simulink model "DTMF"  (Simulink 7.1)
settings: Solver=VariableStepDiscrete  StartTime=0  StopTime=5  RelTol=1e-3
PreLoadFcn:
  | Framesize=256,Fs=8000
undefined symbols (not defined in the file or in its folder): Fs
libraries: dspddes3 x14, dspobslib x3, dspbuff3 x2, commutil2 x2, dspsigops x1, dsparch3 x1, dspswit3 x1, dspwin32 x1
settings Model: Creator=stuartm  LastModifiedBy=jfaing  ExtModeTrigMode=oneshot  ExtModeArmWhenConnect=off  BufferReuse=off
settings DataIOCC: LimitDataPoints=off  SignalLoggingName=sigsOut
settings OptimizationCC: BlockReduction=off  BooleanDataType=off  OptimizeBlockIOStorage=off  BufferReuse=off  EnforceIntegerDowncast=off  ExpressionFolding=off  FoldNonRolledExpr=off  LocalBlockOutputs=off
settings DebuggingCC: SaveWithParameterizedLinksMsg=none  SignalResolutionControl=TryResolveAllWithWarning  SolverPrmCheckMsg=none  MultiTaskDSMMsg=warning  MultiTaskCondExecSysMsg=none  StrictBusMsg=None
settings HardwareCC: TargetUnknown=on
settings RTWCC: IncludeERTFirstTime=on
settings GRTTargetCC: TargetFcnLib=ansi_tfl_tmw.mat

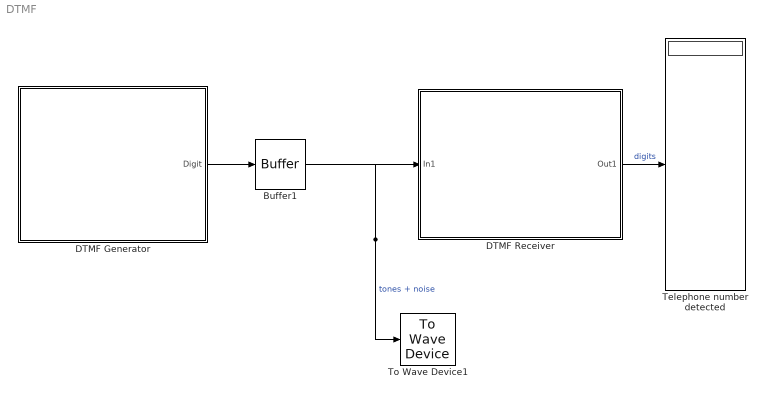
== system DTMF ==
  Buffer1 : dspbuff3/Buffer  N=Framesize  V=0  ic=0
  DTMF Generator : Subsystem
  DTMF Receiver : Subsystem
  Telephone number detected : Display
  To Wave Device1 : dspwin32/To Wave Device  bufDuration=1  determineBufSize=on  userIntBufSize=256  initDelay=0.3  useDefaultDevice=on  userDeviceID=Microsoft RDP Audio Driver  enable24Bit=off
  wires:
  Buffer1/1 -> To Wave Device1/1, DTMF Receiver/1(In1)  "tones + noise"
  DTMF Receiver/1(Out1) -> Telephone number detected/1  "digits"
  DTMF Generator/1(Digit) -> Buffer1/1

== system DTMF/DTMF Generator ==
  Digit to Tone : Subsystem  TreatAsAtomicUnit=on
  Generate telephone number : Subsystem  mask{Number=[1 8 0 0 6 5 3 1 4 1 5], Td=(1/Fs)*256*6}
      mask prompts: Number "Telephone number"; Td "Digit Period (s)"
      mask Display: disp(Number)
  Subtract  1 : Subsystem
  Digit : Outport  OutDataType=sfix(16)  OutScaling=2^0
  wires:
  Generate telephone number/1(Out1) -> Subtract  1/1(In1), Digit to Tone/Enable  "digits"
  Subtract  1/1(Out1) -> Digit to Tone/1(In1)
  Digit to Tone/1(Out1) -> Digit/1

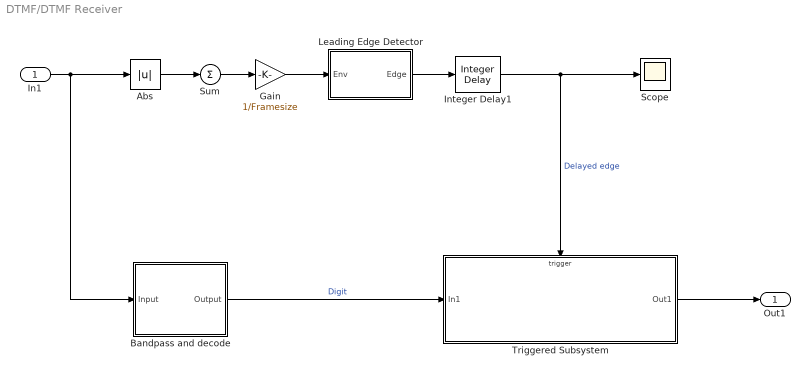
== system DTMF/DTMF Receiver ==
  In1 : Inport  OutDataType=sfix(16)  OutScaling=2^0
  Abs : Abs  SaturateOnIntegerOverflow=on
  Bandpass and decode : Subsystem
  Gain : Gain  Gain=1/Framesize  ParameterDataType=sfix(16)  ParameterScaling=2^0  OutDataType=sfix(16)  OutScaling=2^0  SaturateOnIntegerOverflow=on  OutDataTypeStr=Inherit: Same as input  ParamDataTypeStr=Inherit: Same as input
  Integer Delay1 : dspobslib/Integer Delay  delay=1  ic=0  reset_popup=None
  Leading Edge Detector : Subsystem
  Scope : Scope
  Sum : Sum  Inputs=1  OutDataType=sfix(16)  OutScaling=2^0  SaturateOnIntegerOverflow=on  InputSameDT=on  OutDataTypeStr=Inherit: Same as first input
  Triggered Subsystem : Subsystem  TreatAsAtomicUnit=on
  Out1 : Outport  OutDataType=sfix(16)  OutScaling=2^0
  wires:
  In1/1 -> Abs/1, Bandpass and decode/1(Input)
  Abs/1 -> Sum/1
  Sum/1 -> Gain/1
  Gain/1 -> Leading Edge Detector/1(Env)
  Triggered Subsystem/1(Out1) -> Out1/1
  Integer Delay1/1 -> Scope/1, Triggered Subsystem/Trigger  "Delayed edge"
  Bandpass and decode/1(Output) -> Triggered Subsystem/1(In1)  "Digit"
  Leading Edge Detector/1(Edge) -> Integer Delay1/1

== system DTMF/DTMF Generator/Digit to Tone ==
  In1 : Inport  OutDataType=sfix(16)  OutScaling=2^0
  Enable : EnablePort
  Column Tones 1209Hz 1336Hz 1477Hz : Subsystem
  Column value for digit : Lookup  InputValues=[0 1 2 3 4 5 6 7 8 9 10 11]  Table=[1 0 1 2 0 1 2 0 1 2 0 2]  OutDataType=sfix(16)  OutScaling=2^0  SaturateOnIntegerOverflow=on
  "Row Tones 697Hz 770Hz 852Hz 941Hz " : Subsystem
  Row value for digit : Lookup  InputValues=[0 1 2 3 4 5 6 7 8 9 10 11]  Table=[3 0 0 0 1 1 1 2 2 2 3 3]  OutDataType=sfix(16)  OutScaling=2^0  SaturateOnIntegerOverflow=on
  Sum : Sum  Inputs=|+-  OutDataType=sfix(16)  OutScaling=2^0  SaturateOnIntegerOverflow=on  InputSameDT=on  OutDataTypeStr=Inherit: Same as first input
  Out1 : Outport  OutDataType=sfix(16)  OutScaling=2^0  OutputWhenDisabled=reset  InitialOutput=0
  wires:
  "Row Tones 697Hz 770Hz 852Hz 941Hz "/1(Tone) -> Sum/1
  Column Tones 1209Hz 1336Hz 1477Hz/1(Tone) -> Sum/2
  In1/1 -> Row value for digit/1, Column value for digit/1
  Row value for digit/1 -> "Row Tones 697Hz 770Hz 852Hz 941Hz "/1(Row)
  Column value for digit/1 -> Column Tones 1209Hz 1336Hz 1477Hz/1(Column)
  Sum/1 -> Out1/1

== system DTMF/DTMF Generator/Generate telephone number ==
  Discrete Pulse Generator : DiscretePulseGenerator  SampleTime=Td
  Product : Product  OutDataType=sfix(16)  OutScaling=2^0  SaturateOnIntegerOverflow=on  InputSameDT=on  OutDataTypeStr=Inherit: Same as first input
  Triggered Signal From Workspace1 : dspsigops/Triggered Signal From Workspace  SystemSampleTime=-1  Signal=Number+1  TriggerType=Rising edge  ic=0  SamplesPerFrame=1  OutputAfterFinalValue=Setting to zero
  Out1 : Outport  OutDataType=sfix(16)  OutScaling=2^0
  wires:
  Discrete Pulse Generator/1 -> Product/1, Triggered Signal From Workspace1/Trigger
  Triggered Signal From Workspace1/1 -> Product/2
  Product/1 -> Out1/1

== system DTMF/DTMF Generator/Subtract  1 ==
  In1 : Inport  OutDataType=sfix(16)  OutScaling=2^0
  Constant : Constant  OutDataType=sfix(16)  OutScaling=2^0
  Sum : Sum  Inputs=|+-  OutDataType=sfix(16)  OutScaling=2^0  SaturateOnIntegerOverflow=on  InputSameDT=on  OutDataTypeStr=Inherit: Same as first input
  Out1 : Outport  OutDataType=sfix(16)  OutScaling=2^0
  wires:
  Constant/1 -> Sum/2
  In1/1 -> Sum/1
  Sum/1 -> Out1/1

== system DTMF/DTMF Receiver/Bandpass and decode ==
  Input : Inport  OutDataType=sfix(16)  OutScaling=2^0
  Calculate Digit : Lookup2D  RowIndex=[1:4]  ColumnIndex=[1:3]  Table=[1 2 3;4 5 6;7 8 9;10 0 11]  LookUpMeth=Use Input Nearest  OutDataTypeMode=double  OutDataType=sfix(16)  OutScaling=2^0  OutDataTypeStr=double  SaturateOnIntegerOverflow=on  InputSameDT=on
  Calculate Column : Subsystem
  Calculate Row : Subsystem
  Output : Outport  OutDataType=sfix(16)  OutScaling=2^0
  wires:
  Input/1 -> Calculate Column/1(In1), Calculate Row/1(In1)  "Input Tones"
  Calculate Digit/1 -> Output/1
  Calculate Row/1(Out1) -> Calculate Digit/1
  Calculate Column/1(Out1) -> Calculate Digit/2

== system DTMF/DTMF Receiver/Leading Edge Detector ==
  Env : Inport  OutDataType=sfix(16)  OutScaling=2^0
  Binary To Bipolar : Fcn  Expr=2*u-1
  Constant : Constant  Value=0.5  OutDataType=sfix(16)  OutScaling=2^0
  Direct-Form II Transpose Filter : dsparch3/Direct-Form II Transpose Filter  num=[ones(1,4) -ones(1,4)]  den=1  ic=0
  Edge Detector1 : dspswit3/Edge Detector  SystemSampleTime=-1
  Relational Operator : RelationalOperator  InputSameDT=on
  Rising Edge Start : Fcn  Expr=u>5
  Edge : Outport  OutDataType=sfix(16)  OutScaling=2^0  InitialOutput=0
  wires:
  Edge Detector1/1 -> Edge/1
  Direct-Form II Transpose Filter/1 -> Rising Edge Start/1
  Binary To Bipolar/1 -> Direct-Form II Transpose Filter/1
  Rising Edge Start/1 -> Edge Detector1/1
  Env/1 -> Relational Operator/1
  Constant/1 -> Relational Operator/2
  Relational Operator/1 -> Binary To Bipolar/1

== system DTMF/DTMF Receiver/Triggered Subsystem ==
  In1 : Inport  OutDataType=sfix(16)  OutScaling=2^0
  Trigger : TriggerPort
  Buffer : dspbuff3/Buffer  N=11  V=10  ic=0
  Out1 : Outport  OutDataType=sfix(16)  OutScaling=2^0
  wires:
  In1/1 -> Buffer/1
  Buffer/1 -> Out1/1

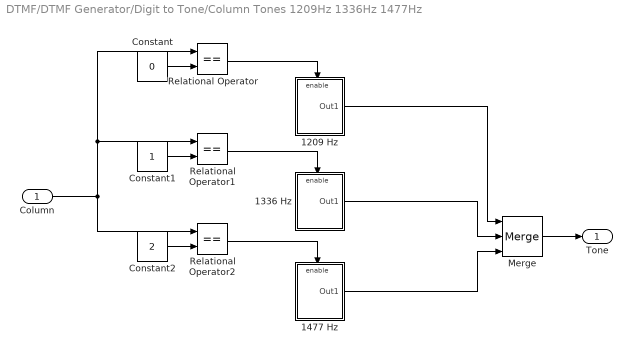
== system DTMF/DTMF Generator/Digit to Tone/Column Tones 1209Hz 1336Hz 1477Hz ==
  Column : Inport  OutDataType=sfix(16)  OutScaling=2^0
  1209 Hz : Subsystem  TreatAsAtomicUnit=on
  1336 Hz : Subsystem  TreatAsAtomicUnit=on
  1477 Hz : Subsystem  TreatAsAtomicUnit=on
  Constant : Constant  Value=0  OutDataType=sfix(16)  OutScaling=2^0
  Constant1 : Constant  OutDataType=sfix(16)  OutScaling=2^0
  Constant2 : Constant  Value=2  OutDataType=sfix(16)  OutScaling=2^0
  Merge : Merge  Inputs=3
  Relational Operator : RelationalOperator  Operator===  InputSameDT=on
  Relational Operator1 : RelationalOperator  Operator===  InputSameDT=on
  Relational Operator2 : RelationalOperator  Operator===  InputSameDT=on
  Tone : Outport  OutDataType=sfix(16)  OutScaling=2^0
  wires:
  Constant2/1 -> Relational Operator2/2
  Constant1/1 -> Relational Operator1/2
  Constant/1 -> Relational Operator/2
  Relational Operator2/1 -> 1477 Hz/Enable
  Relational Operator1/1 -> 1336 Hz/Enable
  Relational Operator/1 -> 1209 Hz/Enable
  Column/1 -> Relational Operator2/1, Relational Operator1/1, Relational Operator/1
  1209 Hz/1(Out1) -> Merge/1
  1336 Hz/1(Out1) -> Merge/2
  1477 Hz/1(Out1) -> Merge/3
  Merge/1 -> Tone/1

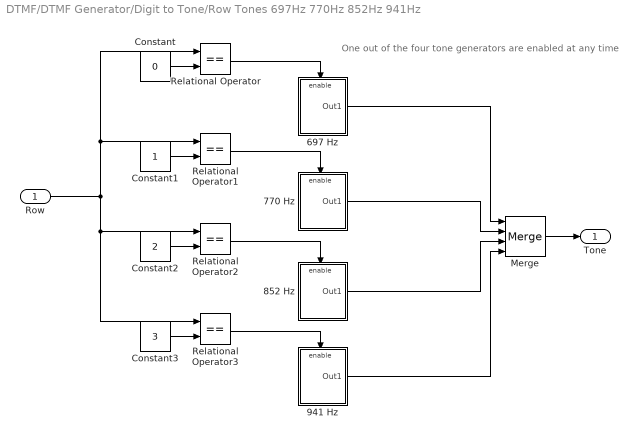
== system DTMF/DTMF Generator/Digit to Tone/Row Tones 697Hz 770Hz 852Hz 941Hz  ==
  note: One out of the four tone generators
      | are enabled at any time
  Row : Inport  OutDataType=sfix(16)  OutScaling=2^0
  697 Hz : Subsystem  TreatAsAtomicUnit=on
  770 Hz : Subsystem  TreatAsAtomicUnit=on
  852 Hz : Subsystem  TreatAsAtomicUnit=on
  941 Hz : Subsystem  TreatAsAtomicUnit=on
  Constant : Constant  Value=0  OutDataType=sfix(16)  OutScaling=2^0
  Constant1 : Constant  OutDataType=sfix(16)  OutScaling=2^0
  Constant2 : Constant  Value=2  OutDataType=sfix(16)  OutScaling=2^0
  Constant3 : Constant  Value=3  OutDataType=sfix(16)  OutScaling=2^0
  Merge : Merge  Inputs=4
  Relational Operator{,1..3} (4 alike) : RelationalOperator  Operator===  InputSameDT=on
  Tone : Outport  OutDataType=sfix(16)  OutScaling=2^0
  wires:
  Constant3/1 -> Relational Operator3/2
  Constant2/1 -> Relational Operator2/2
  Constant1/1 -> Relational Operator1/2
  Constant/1 -> Relational Operator/2
  Relational Operator3/1 -> 941 Hz/Enable
  Relational Operator2/1 -> 852 Hz/Enable
  Relational Operator1/1 -> 770 Hz/Enable
  Relational Operator/1 -> 697 Hz/Enable
  Merge/1 -> Tone/1
  941 Hz/1(Out1) -> Merge/4
  852 Hz/1(Out1) -> Merge/3
  770 Hz/1(Out1) -> Merge/2
  697 Hz/1(Out1) -> Merge/1
  Row/1 -> Relational Operator3/1, Relational Operator2/1, Relational Operator1/1, Relational Operator/1

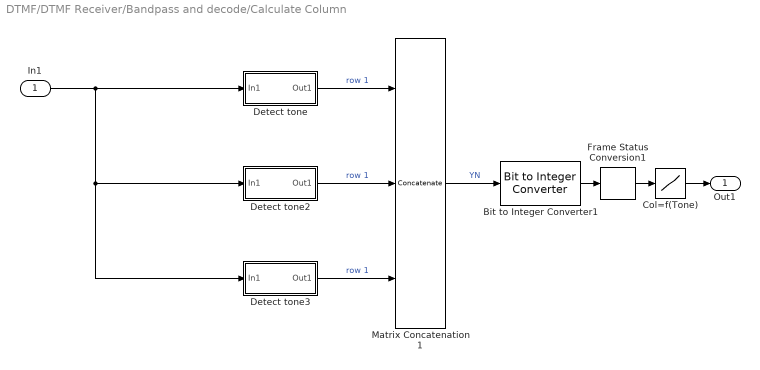
== system DTMF/DTMF Receiver/Bandpass and decode/Calculate Column ==
  In1 : Inport  OutDataType=sfix(16)  OutScaling=2^0
  Bit to Integer Converter1 : commutil2/Bit to Integer Converter  nbits=3  bitOrder=MSB first  signedOutputValues=Unsigned  outDtype=Same as input  outDtypeSigned=Inherit via internal rule
  Col=f(Tone) : Lookup  InputValues=[0:7]  Table=[0 1 2 0 3 0 0 0]  LookUpMeth=Use Input Nearest  OutDataType=sfix(16)  OutScaling=2^0  SaturateOnIntegerOverflow=on
  Detect tone : Subsystem  mask{Fs=Fs, F=1477}
      mask prompts: Fs "Sample Rate (Hz)"; F "Frequency"
      settings: AttributesFormatString=%<F> Hz
  Detect tone2 : Subsystem  mask{Fs=Fs, F=1336}
      mask prompts: Fs "Sample Rate (Hz)"; F "Frequency"
      settings: AttributesFormatString=%<F> Hz
  Detect tone3 : Subsystem  mask{Fs=Fs, F=1209}
      mask prompts: Fs "Sample Rate (Hz)"; F "Frequency"
      settings: AttributesFormatString=%<F> Hz
  Frame Status Conversion1 : dspobslib/Frame Status Conversion  SystemSampleTime=-1  growRefPort=off  outframe=Sample-based
  Matrix Concatenation1 : Concatenate  NumInputs=3  Mode=Multidimensional array
  Out1 : Outport  OutDataType=sfix(16)  OutScaling=2^0
  wires:
  Matrix Concatenation1/1 -> Bit to Integer Converter1/1  "YN"
  Bit to Integer Converter1/1 -> Frame Status Conversion1/1
  Frame Status Conversion1/1 -> Col=f(Tone)/1
  Detect tone/1(Out1) -> Matrix Concatenation1/1  "row 1"
  Detect tone2/1(Out1) -> Matrix Concatenation1/2  "row 1"
  Detect tone3/1(Out1) -> Matrix Concatenation1/3  "row 1"
  In1/1 -> Detect tone2/1(In1), Detect tone3/1(In1), Detect tone/1(In1)
  Col=f(Tone)/1 -> Out1/1

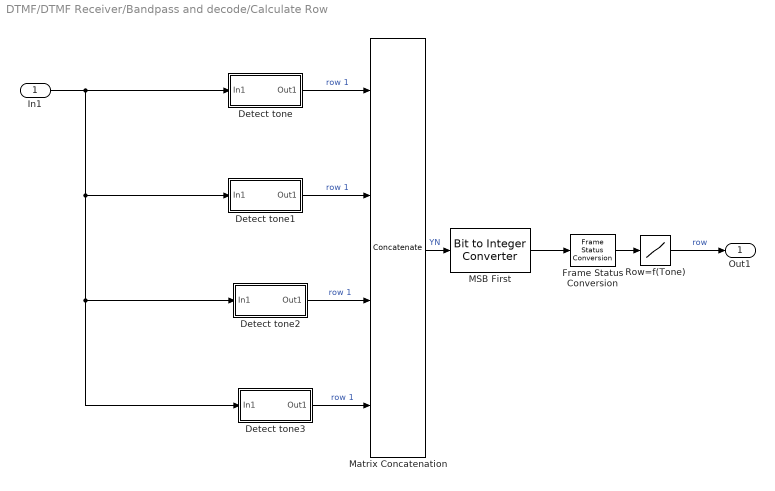
== system DTMF/DTMF Receiver/Bandpass and decode/Calculate Row ==
  In1 : Inport  OutDataType=sfix(16)  OutScaling=2^0
  Detect tone : Subsystem  mask{Fs=Fs, F=941}
      mask prompts: Fs "Sample Rate (Hz)"; F "Frequency"
      settings: AttributesFormatString=%<F> Hz
  Detect tone1 : Subsystem  mask{Fs=Fs, F=852}
      mask prompts: Fs "Sample Rate (Hz)"; F "Frequency"
      settings: AttributesFormatString=%<F> Hz
  Detect tone2 : Subsystem  mask{Fs=Fs, F=770}
      mask prompts: Fs "Sample Rate (Hz)"; F "Frequency"
      settings: AttributesFormatString=%<F> Hz
  Detect tone3 : Subsystem  mask{Fs=Fs, F=697}
      mask prompts: Fs "Sample Rate (Hz)"; F "Frequency"
      settings: AttributesFormatString=%<F> Hz
  Frame Status Conversion : dspobslib/Frame Status Conversion  SystemSampleTime=-1  growRefPort=off  outframe=Sample-based
  MSB First : commutil2/Bit to Integer Converter  nbits=4  bitOrder=MSB first  signedOutputValues=Unsigned  outDtype=Same as input  outDtypeSigned=Inherit via internal rule
  Matrix Concatenation : Concatenate  NumInputs=4  Mode=Multidimensional array
  Row=f(Tone) : Lookup  InputValues=[0:15]  Table=[0 1 2 0 3 0 0 0 4 0 0 0 0 0 0 0]  LookUpMeth=Use Input Nearest  OutDataType=sfix(16)  OutScaling=2^0  SaturateOnIntegerOverflow=on
  Out1 : Outport  OutDataType=sfix(16)  OutScaling=2^0
  wires:
  Detect tone/1(Out1) -> Matrix Concatenation/1  "row 1"
  Matrix Concatenation/1 -> MSB First/1  "YN"
  MSB First/1 -> Frame Status Conversion/1
  Frame Status Conversion/1 -> Row=f(Tone)/1
  Detect tone1/1(Out1) -> Matrix Concatenation/2  "row 1"
  Detect tone2/1(Out1) -> Matrix Concatenation/3  "row 1"
  Detect tone3/1(Out1) -> Matrix Concatenation/4  "row 1"
  In1/1 -> Detect tone/1(In1), Detect tone1/1(In1), Detect tone2/1(In1), Detect tone3/1(In1)
  Row=f(Tone)/1 -> Out1/1  "row"

== system DTMF/DTMF Generator/Digit to Tone/Column Tones 1209Hz 1336Hz 1477Hz/1209 Hz ==
  Enable : EnablePort
  Sine Wave1 : Sin  Frequency=1209*(2*pi)  SampleTime=1/Fs
  Out1 : Outport  OutDataType=sfix(16)  OutScaling=2^0
  wires:
  Sine Wave1/1 -> Out1/1

== system DTMF/DTMF Generator/Digit to Tone/Column Tones 1209Hz 1336Hz 1477Hz/1336 Hz ==
  Enable : EnablePort
  Sine Wave1 : Sin  Frequency=1336*(2*pi)  SampleTime=1/Fs
  Out1 : Outport  OutDataType=sfix(16)  OutScaling=2^0
  wires:
  Sine Wave1/1 -> Out1/1

== system DTMF/DTMF Generator/Digit to Tone/Column Tones 1209Hz 1336Hz 1477Hz/1477 Hz ==
  Enable : EnablePort
  Sine Wave1 : Sin  Frequency=1477*(2*pi)  SampleTime=1/Fs
  Out1 : Outport  OutDataType=sfix(16)  OutScaling=2^0
  wires:
  Sine Wave1/1 -> Out1/1

== system DTMF/DTMF Generator/Digit to Tone/Row Tones 697Hz 770Hz 852Hz 941Hz /697 Hz ==
  Enable : EnablePort
  Sine Wave1 : Sin  Frequency=2*pi*697  SampleTime=1/Fs
  Out1 : Outport  OutDataType=sfix(16)  OutScaling=2^0
  wires:
  Sine Wave1/1 -> Out1/1

== system DTMF/DTMF Generator/Digit to Tone/Row Tones 697Hz 770Hz 852Hz 941Hz /770 Hz ==
  Enable : EnablePort
  Sine Wave1 : Sin  Frequency=2*pi*770  SampleTime=1/Fs
  Out1 : Outport  OutDataType=sfix(16)  OutScaling=2^0
  wires:
  Sine Wave1/1 -> Out1/1

== system DTMF/DTMF Generator/Digit to Tone/Row Tones 697Hz 770Hz 852Hz 941Hz /852 Hz ==
  Enable : EnablePort
  Sine Wave1 : Sin  Frequency=852*(2*pi)  SampleTime=1/Fs
  Out1 : Outport  OutDataType=sfix(16)  OutScaling=2^0
  wires:
  Sine Wave1/1 -> Out1/1

== system DTMF/DTMF Generator/Digit to Tone/Row Tones 697Hz 770Hz 852Hz 941Hz /941 Hz ==
  Enable : EnablePort
  Sine Wave1 : Sin  Frequency=941*(2*pi)  SampleTime=1/Fs
  Out1 : Outport  OutDataType=sfix(16)  OutScaling=2^0
  wires:
  Sine Wave1/1 -> Out1/1

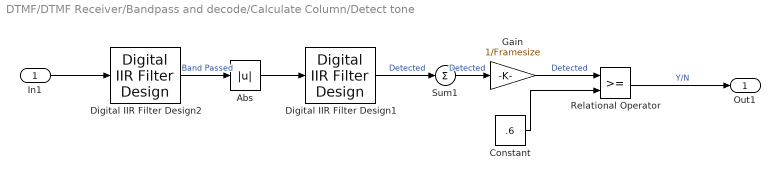
== system DTMF/DTMF Receiver/Bandpass and decode/Calculate Column/Detect tone ==
  In1 : Inport  OutDataType=sfix(16)  OutScaling=2^0
  Abs : Abs  SaturateOnIntegerOverflow=on
  Constant : Constant  Value=.6  OutDataType=sfix(16)  OutScaling=2^0
  Digital IIR Filter Design1 : dspddes3/Digital IIR Filter Design  SystemSampleTime=-1  method=Butterworth  filttype=Lowpass  N=4  Wlo=100/(Fs/2)  Whi=(F+10)/(Fs/2)  Rp=1  Rs=20
  Digital IIR Filter Design2 : dspddes3/Digital IIR Filter Design  SystemSampleTime=-1  method=Chebyshev I  filttype=Bandpass  N=4  Wlo=(F-10)/(Fs/2)  Whi=(F+10)/(Fs/2)  Rp=1  Rs=20
  Gain : Gain  Gain=1/Framesize  ParameterDataType=sfix(16)  ParameterScaling=2^0  OutDataType=sfix(16)  OutScaling=2^0  SaturateOnIntegerOverflow=on  OutDataTypeStr=Inherit: Same as input  ParamDataTypeStr=Inherit: Same as input
  Relational Operator : RelationalOperator  InputSameDT=on
  Sum1 : Sum  Inputs=1  OutDataType=sfix(16)  OutScaling=2^0  SaturateOnIntegerOverflow=on  InputSameDT=on  OutDataTypeStr=Inherit: Same as first input
  Out1 : Outport  OutDataType=sfix(16)  OutScaling=2^0
  wires:
  Digital IIR Filter Design1/1 -> Sum1/1  "Detected"
  Relational Operator/1 -> Out1/1  "Y/N"
  Constant/1 -> Relational Operator/2
  Abs/1 -> Digital IIR Filter Design1/1
  Digital IIR Filter Design2/1 -> Abs/1  "Band Passed"
  In1/1 -> Digital IIR Filter Design2/1
  Sum1/1 -> Gain/1  "Detected"
  Gain/1 -> Relational Operator/1  "Detected"

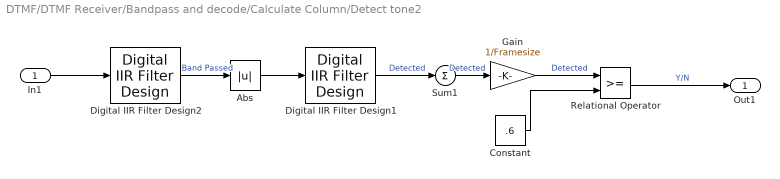
== system DTMF/DTMF Receiver/Bandpass and decode/Calculate Column/Detect tone2 ==
  In1 : Inport  OutDataType=sfix(16)  OutScaling=2^0
  Abs : Abs  SaturateOnIntegerOverflow=on
  Constant : Constant  Value=.6  OutDataType=sfix(16)  OutScaling=2^0
  Digital IIR Filter Design1 : dspddes3/Digital IIR Filter Design  SystemSampleTime=-1  method=Butterworth  filttype=Lowpass  N=4  Wlo=100/(Fs/2)  Whi=(F+10)/(Fs/2)  Rp=1  Rs=20
  Digital IIR Filter Design2 : dspddes3/Digital IIR Filter Design  SystemSampleTime=-1  method=Chebyshev I  filttype=Bandpass  N=4  Wlo=(F-10)/(Fs/2)  Whi=(F+10)/(Fs/2)  Rp=1  Rs=20
  Gain : Gain  Gain=1/Framesize  ParameterDataType=sfix(16)  ParameterScaling=2^0  OutDataType=sfix(16)  OutScaling=2^0  SaturateOnIntegerOverflow=on  OutDataTypeStr=Inherit: Same as input  ParamDataTypeStr=Inherit: Same as input
  Relational Operator : RelationalOperator  InputSameDT=on
  Sum1 : Sum  Inputs=1  OutDataType=sfix(16)  OutScaling=2^0  SaturateOnIntegerOverflow=on  InputSameDT=on  OutDataTypeStr=Inherit: Same as first input
  Out1 : Outport  OutDataType=sfix(16)  OutScaling=2^0
  wires:
  Gain/1 -> Relational Operator/1  "Detected"
  Sum1/1 -> Gain/1  "Detected"
  In1/1 -> Digital IIR Filter Design2/1
  Digital IIR Filter Design2/1 -> Abs/1  "Band Passed"
  Abs/1 -> Digital IIR Filter Design1/1
  Constant/1 -> Relational Operator/2
  Relational Operator/1 -> Out1/1  "Y/N"
  Digital IIR Filter Design1/1 -> Sum1/1  "Detected"

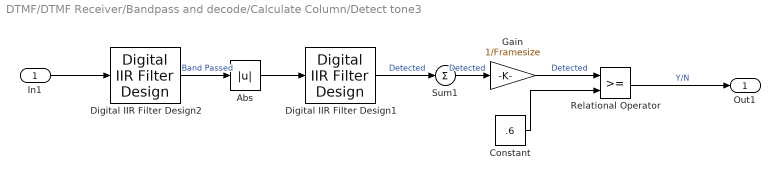
== system DTMF/DTMF Receiver/Bandpass and decode/Calculate Column/Detect tone3 ==
  In1 : Inport  OutDataType=sfix(16)  OutScaling=2^0
  Abs : Abs  SaturateOnIntegerOverflow=on
  Constant : Constant  Value=.6  OutDataType=sfix(16)  OutScaling=2^0
  Digital IIR Filter Design1 : dspddes3/Digital IIR Filter Design  SystemSampleTime=-1  method=Butterworth  filttype=Lowpass  N=4  Wlo=100/(Fs/2)  Whi=(F+10)/(Fs/2)  Rp=1  Rs=20
  Digital IIR Filter Design2 : dspddes3/Digital IIR Filter Design  SystemSampleTime=-1  method=Chebyshev I  filttype=Bandpass  N=4  Wlo=(F-10)/(Fs/2)  Whi=(F+10)/(Fs/2)  Rp=1  Rs=20
  Gain : Gain  Gain=1/Framesize  ParameterDataType=sfix(16)  ParameterScaling=2^0  OutDataType=sfix(16)  OutScaling=2^0  SaturateOnIntegerOverflow=on  OutDataTypeStr=Inherit: Same as input  ParamDataTypeStr=Inherit: Same as input
  Relational Operator : RelationalOperator  InputSameDT=on
  Sum1 : Sum  Inputs=1  OutDataType=sfix(16)  OutScaling=2^0  SaturateOnIntegerOverflow=on  InputSameDT=on  OutDataTypeStr=Inherit: Same as first input
  Out1 : Outport  OutDataType=sfix(16)  OutScaling=2^0
  wires:
  Digital IIR Filter Design1/1 -> Sum1/1  "Detected"
  Relational Operator/1 -> Out1/1  "Y/N"
  Constant/1 -> Relational Operator/2
  Abs/1 -> Digital IIR Filter Design1/1
  Digital IIR Filter Design2/1 -> Abs/1  "Band Passed"
  In1/1 -> Digital IIR Filter Design2/1
  Sum1/1 -> Gain/1  "Detected"
  Gain/1 -> Relational Operator/1  "Detected"

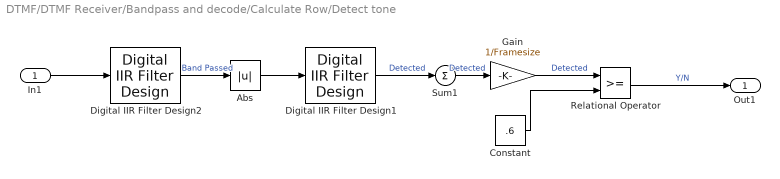
== system DTMF/DTMF Receiver/Bandpass and decode/Calculate Row/Detect tone ==
  In1 : Inport  OutDataType=sfix(16)  OutScaling=2^0
  Abs : Abs  SaturateOnIntegerOverflow=on
  Constant : Constant  Value=.6  OutDataType=sfix(16)  OutScaling=2^0
  Digital IIR Filter Design1 : dspddes3/Digital IIR Filter Design  SystemSampleTime=-1  method=Butterworth  filttype=Lowpass  N=4  Wlo=100/(Fs/2)  Whi=(F+10)/(Fs/2)  Rp=1  Rs=20
  Digital IIR Filter Design2 : dspddes3/Digital IIR Filter Design  SystemSampleTime=-1  method=Chebyshev I  filttype=Bandpass  N=4  Wlo=(F-10)/(Fs/2)  Whi=(F+10)/(Fs/2)  Rp=1  Rs=20
  Gain : Gain  Gain=1/Framesize  ParameterDataType=sfix(16)  ParameterScaling=2^0  OutDataType=sfix(16)  OutScaling=2^0  SaturateOnIntegerOverflow=on  OutDataTypeStr=Inherit: Same as input  ParamDataTypeStr=Inherit: Same as input
  Relational Operator : RelationalOperator  InputSameDT=on
  Sum1 : Sum  Inputs=1  OutDataType=sfix(16)  OutScaling=2^0  SaturateOnIntegerOverflow=on  InputSameDT=on  OutDataTypeStr=Inherit: Same as first input
  Out1 : Outport  OutDataType=sfix(16)  OutScaling=2^0
  wires:
  Gain/1 -> Relational Operator/1  "Detected"
  Sum1/1 -> Gain/1  "Detected"
  In1/1 -> Digital IIR Filter Design2/1
  Digital IIR Filter Design2/1 -> Abs/1  "Band Passed"
  Abs/1 -> Digital IIR Filter Design1/1
  Constant/1 -> Relational Operator/2
  Relational Operator/1 -> Out1/1  "Y/N"
  Digital IIR Filter Design1/1 -> Sum1/1  "Detected"

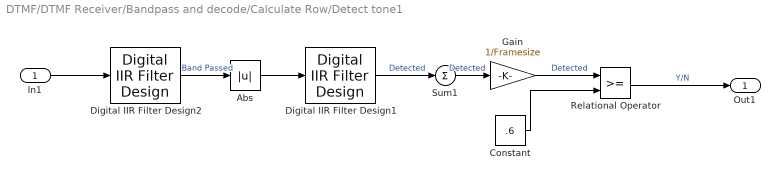
== system DTMF/DTMF Receiver/Bandpass and decode/Calculate Row/Detect tone1 ==
  In1 : Inport  OutDataType=sfix(16)  OutScaling=2^0
  Abs : Abs  SaturateOnIntegerOverflow=on
  Constant : Constant  Value=.6  OutDataType=sfix(16)  OutScaling=2^0
  Digital IIR Filter Design1 : dspddes3/Digital IIR Filter Design  SystemSampleTime=-1  method=Butterworth  filttype=Lowpass  N=4  Wlo=100/(Fs/2)  Whi=(F+10)/(Fs/2)  Rp=1  Rs=20
  Digital IIR Filter Design2 : dspddes3/Digital IIR Filter Design  SystemSampleTime=-1  method=Chebyshev I  filttype=Bandpass  N=4  Wlo=(F-10)/(Fs/2)  Whi=(F+10)/(Fs/2)  Rp=1  Rs=20
  Gain : Gain  Gain=1/Framesize  ParameterDataType=sfix(16)  ParameterScaling=2^0  OutDataType=sfix(16)  OutScaling=2^0  SaturateOnIntegerOverflow=on  OutDataTypeStr=Inherit: Same as input  ParamDataTypeStr=Inherit: Same as input
  Relational Operator : RelationalOperator  InputSameDT=on
  Sum1 : Sum  Inputs=1  OutDataType=sfix(16)  OutScaling=2^0  SaturateOnIntegerOverflow=on  InputSameDT=on  OutDataTypeStr=Inherit: Same as first input
  Out1 : Outport  OutDataType=sfix(16)  OutScaling=2^0
  wires:
  Digital IIR Filter Design1/1 -> Sum1/1  "Detected"
  Relational Operator/1 -> Out1/1  "Y/N"
  Constant/1 -> Relational Operator/2
  Abs/1 -> Digital IIR Filter Design1/1
  Digital IIR Filter Design2/1 -> Abs/1  "Band Passed"
  In1/1 -> Digital IIR Filter Design2/1
  Sum1/1 -> Gain/1  "Detected"
  Gain/1 -> Relational Operator/1  "Detected"

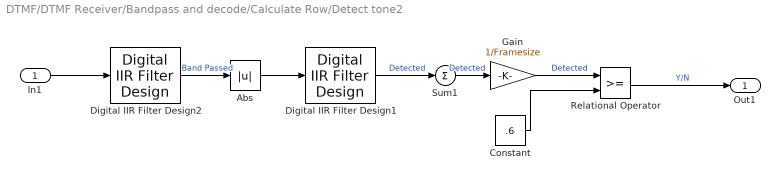
== system DTMF/DTMF Receiver/Bandpass and decode/Calculate Row/Detect tone2 ==
  In1 : Inport  OutDataType=sfix(16)  OutScaling=2^0
  Abs : Abs  SaturateOnIntegerOverflow=on
  Constant : Constant  Value=.6  OutDataType=sfix(16)  OutScaling=2^0
  Digital IIR Filter Design1 : dspddes3/Digital IIR Filter Design  SystemSampleTime=-1  method=Butterworth  filttype=Lowpass  N=4  Wlo=100/(Fs/2)  Whi=(F+10)/(Fs/2)  Rp=1  Rs=20
  Digital IIR Filter Design2 : dspddes3/Digital IIR Filter Design  SystemSampleTime=-1  method=Chebyshev I  filttype=Bandpass  N=4  Wlo=(F-10)/(Fs/2)  Whi=(F+10)/(Fs/2)  Rp=1  Rs=20
  Gain : Gain  Gain=1/Framesize  ParameterDataType=sfix(16)  ParameterScaling=2^0  OutDataType=sfix(16)  OutScaling=2^0  SaturateOnIntegerOverflow=on  OutDataTypeStr=Inherit: Same as input  ParamDataTypeStr=Inherit: Same as input
  Relational Operator : RelationalOperator  InputSameDT=on
  Sum1 : Sum  Inputs=1  OutDataType=sfix(16)  OutScaling=2^0  SaturateOnIntegerOverflow=on  InputSameDT=on  OutDataTypeStr=Inherit: Same as first input
  Out1 : Outport  OutDataType=sfix(16)  OutScaling=2^0
  wires:
  Gain/1 -> Relational Operator/1  "Detected"
  Sum1/1 -> Gain/1  "Detected"
  In1/1 -> Digital IIR Filter Design2/1
  Digital IIR Filter Design2/1 -> Abs/1  "Band Passed"
  Abs/1 -> Digital IIR Filter Design1/1
  Constant/1 -> Relational Operator/2
  Relational Operator/1 -> Out1/1  "Y/N"
  Digital IIR Filter Design1/1 -> Sum1/1  "Detected"

== system DTMF/DTMF Receiver/Bandpass and decode/Calculate Row/Detect tone3 ==
  In1 : Inport  OutDataType=sfix(16)  OutScaling=2^0
  Abs : Abs  SaturateOnIntegerOverflow=on
  Constant : Constant  Value=.6  OutDataType=sfix(16)  OutScaling=2^0
  Digital IIR Filter Design1 : dspddes3/Digital IIR Filter Design  SystemSampleTime=-1  method=Butterworth  filttype=Lowpass  N=4  Wlo=100/(Fs/2)  Whi=(F+10)/(Fs/2)  Rp=1  Rs=20
  Digital IIR Filter Design2 : dspddes3/Digital IIR Filter Design  SystemSampleTime=-1  method=Chebyshev I  filttype=Bandpass  N=4  Wlo=(F-10)/(Fs/2)  Whi=(F+10)/(Fs/2)  Rp=1  Rs=20
  Gain : Gain  Gain=1/Framesize  ParameterDataType=sfix(16)  ParameterScaling=2^0  OutDataType=sfix(16)  OutScaling=2^0  SaturateOnIntegerOverflow=on  OutDataTypeStr=Inherit: Same as input  ParamDataTypeStr=Inherit: Same as input
  Relational Operator : RelationalOperator  InputSameDT=on
  Sum1 : Sum  Inputs=1  OutDataType=sfix(16)  OutScaling=2^0  SaturateOnIntegerOverflow=on  InputSameDT=on  OutDataTypeStr=Inherit: Same as first input
  Out1 : Outport  OutDataType=sfix(16)  OutScaling=2^0
  wires:
  Digital IIR Filter Design1/1 -> Sum1/1  "Detected"
  Relational Operator/1 -> Out1/1  "Y/N"
  Constant/1 -> Relational Operator/2
  Abs/1 -> Digital IIR Filter Design1/1
  Digital IIR Filter Design2/1 -> Abs/1  "Band Passed"
  In1/1 -> Digital IIR Filter Design2/1
  Sum1/1 -> Gain/1  "Detected"
  Gain/1 -> Relational Operator/1  "Detected"
